simulink model "WholeSystemSimulation"  (R2024b)
settings: Solver=FixedStepAuto  StartTime=0.0  StopTime=3  FixedStep=1/executionRate  MaxStep=0.01  RelTol=1e-3
values from neighbouring files (symbols this model uses):
  executionRate = 5*ADC_SamplingRate    (= 25000)    [parameters.m]
undefined symbols (not defined in the file or in its folder): Batt, VCCS
libraries: fl_lib x15, spsFourierLib x4, nesl_utility x4, simulink_extras x2, ee_lib x1
settings Model: SnapshotBufferSize=100  SnapshotInterval=100  Creator=JesseJabezArendse  LastModifiedBy=JesseJabezArendse
settings SolverCC: MaxConsecutiveMinStep=1000  ShapePreserveControl=EnableAll  ZeroCrossControl=EnableAll  ZeroCrossAlgorithm=Adaptive
settings DebuggingCC: MaskedZcDiagnostic=none  IgnoredZcDiagnostic=none
settings RTWCC: GPUComputeCapability=3.5
settings SimscapeCC: ExplicitSolverDiagnosticOptions=none  SimscapeCompileComponentReuse=on

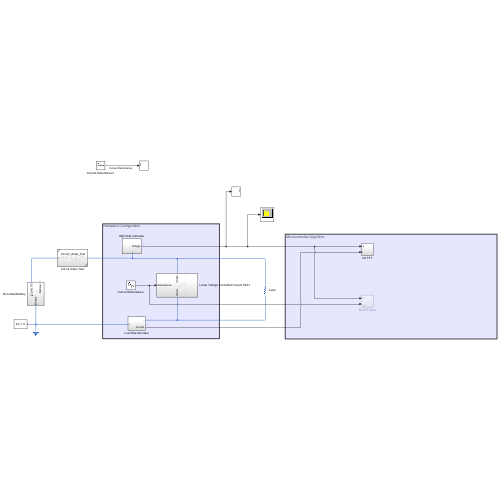
[thumbnail: Simulink's stored preview of the top-level diagram]
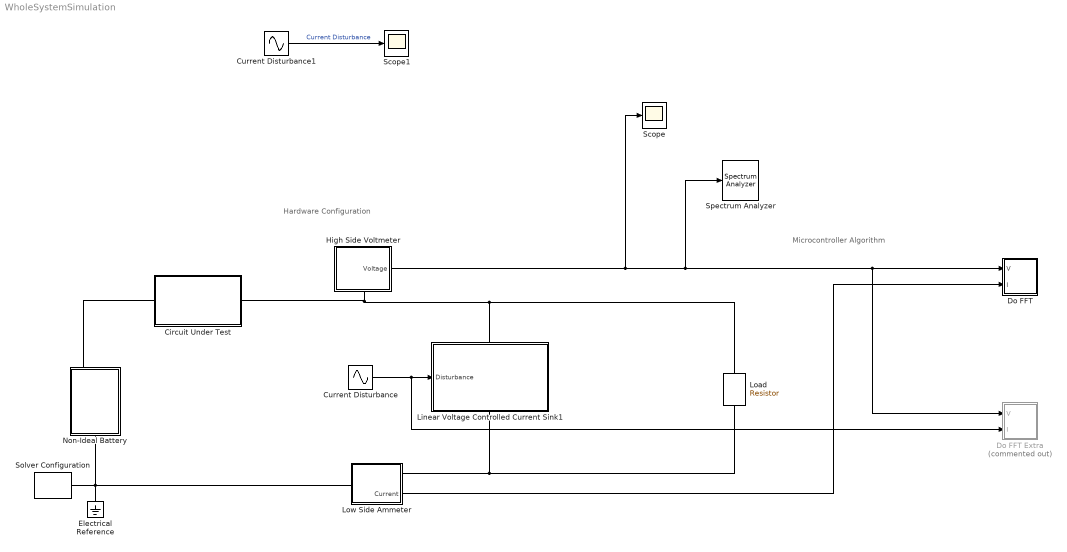
== system WholeSystemSimulation ==
  note: Microcontroller Algorithm
  note: Hardware Configuration
  Circuit Under Test : Subsystem  ReferencedSubsystem=Circuit_Under_Test
  Current Disturbance : Sin  Amplitude=VCCS.Ic/2  Bias=VCCS.Ic/2  Frequency=2*pi*1000  SampleTime=0
  Current Disturbance1 : Sin  Amplitude=VCCS.Ic/2  Bias=VCCS.Ic/2  Frequency=2*pi*1  Phase=-pi/2  SampleTime=0
  Do FFT : Subsystem
  Do FFT Extra : Subsystem  Commented=on
  Electrical Reference : fl_lib/Electrical/Electrical Elements/Electrical Reference
  High Side Voltmeter : Subsystem
      settings: PortSchema="{\"entries\":[{\"content\":{\"sides\":[{\"content\":{\"connectorIds\":[\"LConn1\"]},\"type\":\"ConnectorPlacement.EquallySpacedRectSide\",\"uuid\":\"dc1b0a43-9892-4e76-b578-c6766fff3160\"},{\"content\":{\"side\":\"RIGHT\"},\"type\":\"ConnectorPlacement.EquallySpacedRectSide\",\"uuid\":\"9def735b-7f91-462a-b4cf-02dbc37cb50d\"},{\"content\":{\"connectorIds\":[\"Out1\"],\"side\":\"TOP\"},\"type\":\"ConnectorPlacement.EquallySpacedRectSide\",\"uuid\":\"48b0b69b-e7ce-41ab-9991-9433c11ca6b3\"}]},\"type\":\"ConnectorPlacement.EquallySpacedConnector\",\"uuid\":\"81e0c23a-938e-4893-99ad-7cd29a79d819\"}],\"packageUris\":[\"http://schema.mathworks.com/mf0/Connector/R2020b\"],\"version\":\"1.0\"}"
  Linear Voltage Controlled Current Sink1 : Subsystem
      settings: PortSchema="{\"entries\":[{\"content\":{\"sides\":[{\"content\":{\"connectorIds\":[\"In1\"]},\"type\":\"ConnectorPlacement.EquallySpacedRectSide\",\"uuid\":\"18d529a9-1cf8-4422-88d7-d8552fbc69b1\"},{\"content\":{\"side\":\"RIGHT\"},\"type\":\"ConnectorPlacement.EquallySpacedRectSide\",\"uuid\":\"d099dce7-fb34-4cde-a1aa-9938a0a6f030\"},{\"content\":{\"connectorIds\":[\"LConn1\"],\"side\":\"TOP\"},\"type\":\"ConnectorPlacement.EquallySpacedRectSide\",\"uuid\":\"f8047e6b-d66f-4a7e-8493-e8033d6b44b9\"},{\"content\":{\"connectorIds\":[\"RConn1\"],\"side\":\"BOTTOM\"},\"type\":\"ConnectorPlacement.EquallySpacedRectSide\",\"uuid\":\"82df79ce-b48a-4c65-8b98-c5c94047aaf0\"}]},\"type\":\"ConnectorPlacement.EquallySpacedConnector\",\"uuid\":\"b1df41be-ee9b-457e-b8ab-8cc4e6bfe837\"}],\"packageUris\":[\"http://schema.mathworks.com/mf0/Connector/R2020b\"],\"version\":\"1.0\"}"
  Load : fl_lib/Electrical/Electrical Elements/Resistor  R=15 Ohm  i_specify=off  i_priority=None  i=0 A  i_nominal_specify=off  i_nominal_value=1  i_nominal_unit=A  v_specify=off  v_priority=None  v=0 V  v_nominal_specify=off  v_nominal_value=1  v_nominal_unit=V
  Low Side Ammeter : Subsystem
      settings: PortSchema="{\"entries\":[{\"content\":{\"sides\":[{\"content\":{\"connectorIds\":[\"LConn1\"]},\"type\":\"ConnectorPlacement.EquallySpacedRectSide\",\"uuid\":\"b46022f5-6657-4f49-902e-44a46ebfa2aa\"},{\"content\":{\"connectorIds\":[\"RConn1\",\"Out1\"],\"side\":\"RIGHT\"},\"type\":\"ConnectorPlacement.EquallySpacedRectSide\",\"uuid\":\"78fe3371-6c6c-498b-a57a-7222f53b6f75\"},{\"content\":{\"side\":\"TOP\"},\"type\":\"ConnectorPlacement.EquallySpacedRectSide\",\"uuid\":\"f620f906-e4ba-4bb0-90eb-5c83cecaa9b0\"}]},\"type\":\"ConnectorPlacement.EquallySpacedConnector\",\"uuid\":\"c8c374b0-8252-47d0-a7d3-288c91bf26d8\"}],\"packageUris\":[\"http://schema.mathworks.com/mf0/Connector/R2020b\"],\"version\":\"1.0\"}"
  Non-Ideal Battery : Subsystem
  Scope : Scope
  Scope1 : Scope
  Solver Configuration : nesl_utility/Solver Configuration  PhysicalDomain=network_engine_domain  SubClassName=solver  LeftPortType=input  RightPortType=generic  Tones=[]  Harmonics=[]  SimulateNoise=off  Profile=off  UseLocalSampling=off  EnableSwitchedLinearOptims=on  FrequencyDomain=off  UseCCode=off  RelTol=0.001  AbsTol=0.001  MinStep=1e-09  ToWorkspace=off  RevertToSquareIcSolve=off  NumHomotopyIterations=100  PhasorMode=off  PhasorModeNumHarmonics=1  ConsistencySolver=NEWTON_XTOL_AFTER_FTOL  IndexReductionMethod=None  DoDC=on  ResidualTolerance=1e-09  ConsistencyTolSource=LOCAL  ConsistencyAbsTol=0.001  ConsistencyRelTol=0.001  ConsistencyTolFactor=0.00001  UseLocalSolver=on  LocalSolverChoice=NE_BACKWARD_EULER_ADVANCER  ResolveIndetEquations=on  FunctionEvalNumThread=1  LocalSolverSampleTime=1/executionRate  DoFixedCost=off  MaxNonlinIter=3  MaxModeIter=2  ComputeImpulses=off  ImpulseIterations=2  LinearAlgebra=auto  LinearAlgebraNumThread=0  EquationFormulation=NE_TIME_EF  DelaysMemoryBudget=1024  AutomaticFiltering=off  FilteringTimeConstant=0.001  PartitionStorageMethod=AS_NEEDED  PartitionMemoryBudget=1024  PartitionMethod=ROBUST  MultibodyUseLocalSolver=off  MultibodyLocalSolverChoice=ODE1  MultibodyLocalSolverSampleTime=0.001
  Spectrum Analyzer : SpectrumAnalyzer  WindowPosition=[-276.000000,-288.000000,1536.000000,792.000000,]  ScopeFrameLocation=window  SampleRateSource=Property  SampleRate=50000  WindowInvariantSamplesPerUpdate=on  Span=50000  StartFrequency=-25000  StopFrequency=25000  YLimits=[-122.6326188,59.51523193]  ShowLegend=on
  wires:
  Current Disturbance/1 -> Do FFT Extra/2(I), Linear Voltage Controlled Current Sink1/1(Disturbance)
  High Side Voltmeter/1(Voltage) -> Scope/1, Spectrum Analyzer/1, Do FFT Extra/1(V), Do FFT/1(V)
  Low Side Ammeter/1(Current) -> Do FFT/2(I)
  Current Disturbance1/1 -> Scope1/1  "Current Disturbance"
  connections:
  Solver Configuration/RConn1 -- Low Side Ammeter/LConn1 -- Non-Ideal Battery/RConn1 -- Electrical Reference/LConn1
  High Side Voltmeter/LConn1 -- Linear Voltage Controlled Current Sink1/LConn1 -- Load/LConn1 -- Circuit Under Test/RConn1
  Low Side Ammeter/RConn1 -- Linear Voltage Controlled Current Sink1/RConn1 -- Load/RConn1
  Non-Ideal Battery/LConn1 -- Circuit Under Test/LConn1

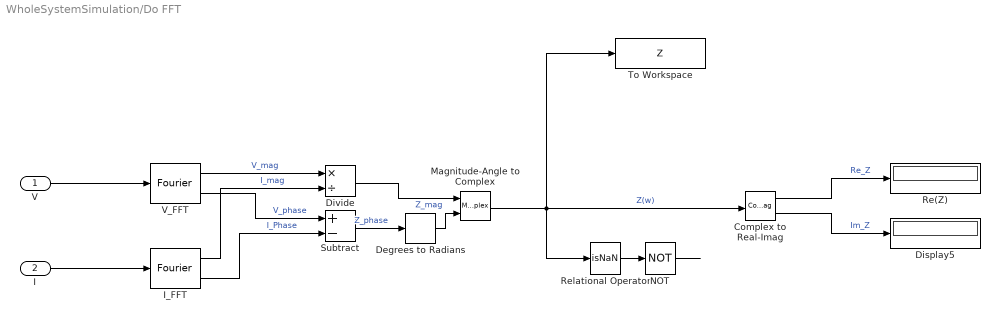
== system WholeSystemSimulation/Do FFT ==
  V : Inport
  I : Inport  Port=2
  Complex to Real-Imag : ComplexToRealImag
  Degrees to Radians : simulink_extras/Transformations/Degrees to Radians
  Display5 : Display
  Divide : Product  Inputs=*/
  I_FFT : spsFourierLib/Fourier  Freq=selectedFreq  n=1  InInit=[0, 0]  Ts=0
  Magnitude-Angle to Complex : MagnitudeAngleToComplex
  NOT : Logic  Operator=NOT  IconShape=distinctive  AllPortsSameDT=off  OutDataTypeStr=boolean
  Re(Z) : Display
  Relational Operator : RelationalOperator  Operator=isNaN  OutDataTypeStr=boolean  RndMeth=Simplest  InputSameDT=off
  Subtract : Sum  Inputs=+-
  To Workspace : ToWorkspace  VariableName=Z  SampleTime=-1
  V_FFT : spsFourierLib/Fourier  Freq=selectedFreq  n=1  InInit=[0, 0]  Ts=0
  wires:
  V_FFT/1 -> Divide/1  "V_mag"
  Degrees to Radians/1 -> Magnitude-Angle to Complex/2
  Magnitude-Angle to Complex/1 -> To Workspace/1, Complex to Real-Imag/1, Relational Operator/1  "Z(w)"
  Complex to Real-Imag/1 -> Re(Z)/1  "Re_Z"
  V_FFT/2 -> Subtract/1  "V_phase"
  I_FFT/2 -> Subtract/2  "I_Phase"
  Complex to Real-Imag/2 -> Display5/1  "Im_Z"
  Subtract/1 -> Degrees to Radians/1  "Z_phase"
  I_FFT/1 -> Divide/2  "I_mag"
  Divide/1 -> Magnitude-Angle to Complex/1  "Z_mag"
  I/1 -> I_FFT/1
  V/1 -> V_FFT/1
  Relational Operator/1 -> NOT/1
  NOT/1 -> ?

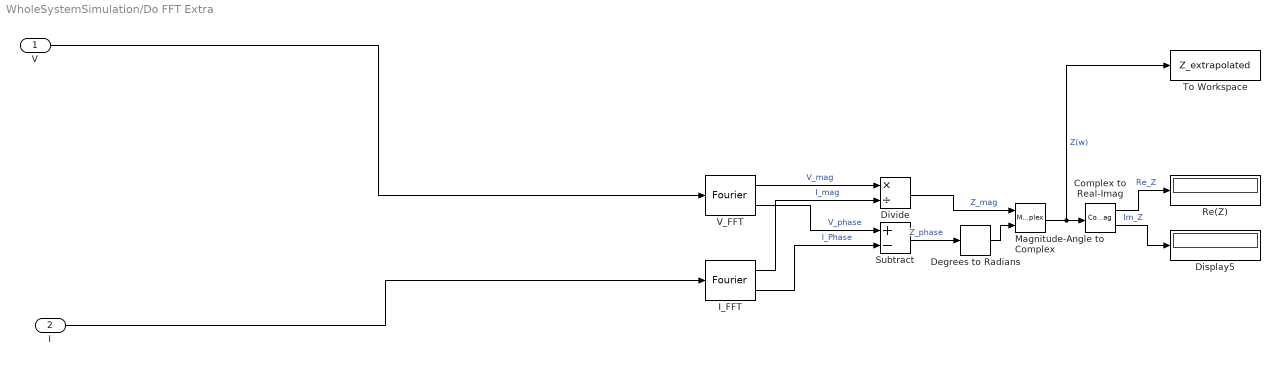
== system WholeSystemSimulation/Do FFT Extra ==
  V : Inport
  I : Inport  Port=2
  Complex to Real-Imag : ComplexToRealImag
  Degrees to Radians : simulink_extras/Transformations/Degrees to Radians
  Display5 : Display
  Divide : Product  Inputs=*/
  I_FFT : spsFourierLib/Fourier  Freq=selectedFreq  n=1  InInit=[0, 0]  Ts=0
  Magnitude-Angle to Complex : MagnitudeAngleToComplex
  Re(Z) : Display
  Subtract : Sum  Inputs=+-
  To Workspace : ToWorkspace  VariableName=Z_extrapolated  SampleTime=-1
  V_FFT : spsFourierLib/Fourier  Freq=selectedFreq  n=1  InInit=[0, 0]  Ts=0
  wires:
  V/1 -> V_FFT/1
  I/1 -> I_FFT/1
  Divide/1 -> Magnitude-Angle to Complex/1  "Z_mag"
  I_FFT/1 -> Divide/2  "I_mag"
  Subtract/1 -> Degrees to Radians/1  "Z_phase"
  Complex to Real-Imag/2 -> Display5/1  "Im_Z"
  I_FFT/2 -> Subtract/2  "I_Phase"
  V_FFT/2 -> Subtract/1  "V_phase"
  Complex to Real-Imag/1 -> Re(Z)/1  "Re_Z"
  Magnitude-Angle to Complex/1 -> Complex to Real-Imag/1, To Workspace/1  "Z(w)"
  Degrees to Radians/1 -> Magnitude-Angle to Complex/2
  V_FFT/1 -> Divide/1  "V_mag"

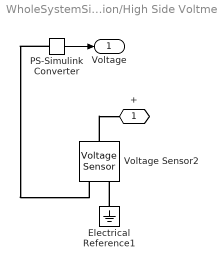
== system WholeSystemSimulation/High Side Voltmeter ==
  Electrical Reference1 : fl_lib/Electrical/Electrical Elements/Electrical Reference
  PS-Simulink Converter : nesl_utility/PS-Simulink Converter  PhysicalDomain=network_engine_domain  SubClassName=ps_output  LeftPortType=input  RightPortType=output  PseudoPeriodic=off  Frequencies=[]  VectorFormat=inherit  Unit=inherit  AffineConversion=off
  Voltage Sensor2 : fl_lib/Electrical/Electrical Sensors/Voltage Sensor
  + : PMIOPort  Side=Left
  Voltage : Outport
  wires:
  PS-Simulink Converter/1 -> Voltage/1
  connections:
  Electrical Reference1/LConn1 -- Voltage Sensor2/RConn2
  PS-Simulink Converter/LConn1 -- Voltage Sensor2/RConn1
  Voltage Sensor2/LConn1 -- +/RConn1

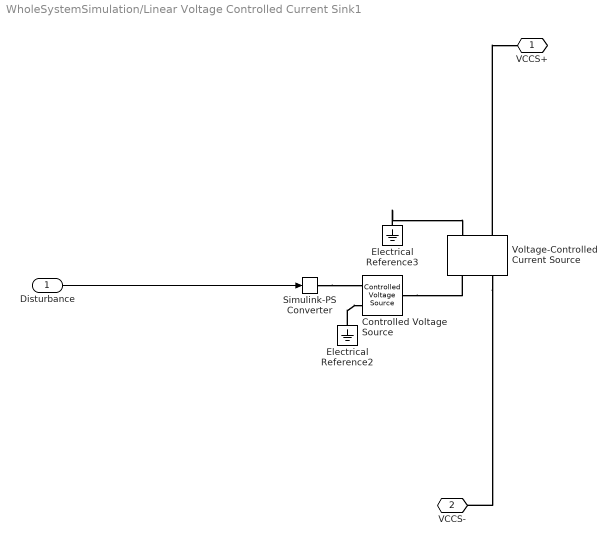
== system WholeSystemSimulation/Linear Voltage Controlled Current Sink1 ==
  Disturbance : Inport
  Controlled Voltage Source : fl_lib/Electrical/Electrical Sources/Controlled Voltage Source
  Electrical Reference2 : fl_lib/Electrical/Electrical Elements/Electrical Reference
  Electrical Reference3 : fl_lib/Electrical/Electrical Elements/Electrical Reference
  Simulink-PS Converter : nesl_utility/Simulink-PS Converter  PhysicalDomain=network_engine_domain  SubClassName=ps_input  LeftPortType=input  RightPortType=output  PseudoPeriodic=off  Frequencies=[]  NoiseDistribution=none  NoiseParameters=[]  Unit=1  AffineConversion=off  FilteringAndDerivatives=provide  SimscapeFilterOrder=1  InputFilterTimeConstant=0.001  UdotUserProvided=0
  Voltage-Controlled Current Source : fl_lib/Electrical/Electrical Sources/Voltage-Controlled Current Source  K=1 1/Ohm  v1_specify=off  v1_priority=None  v1=0 V  v1_nominal_specify=off  v1_nominal_value=1  v1_nominal_unit=V  i2_specify=off  i2_priority=None  i2=0 A  i2_nominal_specify=off  i2_nominal_value=1  i2_nominal_unit=A
      settings: InternalSimscapePortConfiguration="{\"Bottom\":[],\"Left\":[{\"id\":\"p1\",\"label\":\"+\",\"type\":\"foundation.electrical.electrical\"},{\"id\":\"head\",\"label\":\"\",\"type\":\"foundation.electrical.electrical\"}],\"Right\":[{\"id\":\"n1\",\"label\":\"-\",\"type\":\"foundation.electrical.electrical\"},{\"id\":\"tail\",\"label\":\"\",\"type\":\"foundation.electrical.electrical\"}],\"Top\":[]}"
  VCCS+ : PMIOPort  Side=Left
  VCCS- : PMIOPort  Port=2  Side=Right
  wires:
  Disturbance/1 -> Simulink-PS Converter/1
  connections:
  Electrical Reference2/LConn1 -- Controlled Voltage Source/RConn2
  Voltage-Controlled Current Source/RConn2 -- VCCS+/RConn1
  Voltage-Controlled Current Source/LConn2 -- VCCS-/RConn1
  Simulink-PS Converter/RConn1 -- Controlled Voltage Source/RConn1
  Electrical Reference3/LConn1 -- Voltage-Controlled Current Source/RConn1
  Controlled Voltage Source/LConn1 -- Voltage-Controlled Current Source/LConn1

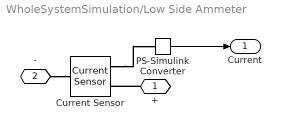
== system WholeSystemSimulation/Low Side Ammeter ==
  Current Sensor : fl_lib/Electrical/Electrical Sensors/Current Sensor
  PS-Simulink Converter : nesl_utility/PS-Simulink Converter  PhysicalDomain=network_engine_domain  SubClassName=ps_output  LeftPortType=input  RightPortType=output  PseudoPeriodic=off  Frequencies=[]  VectorFormat=inherit  Unit=inherit  AffineConversion=off
  + : PMIOPort  Side=Left
  - : PMIOPort  Port=2  Side=Right
  Current : Outport
  wires:
  PS-Simulink Converter/1 -> Current/1
  connections:
  Current Sensor/RConn1 -- PS-Simulink Converter/LConn1
  +/RConn1 -- Current Sensor/RConn2
  -/RConn1 -- Current Sensor/LConn1

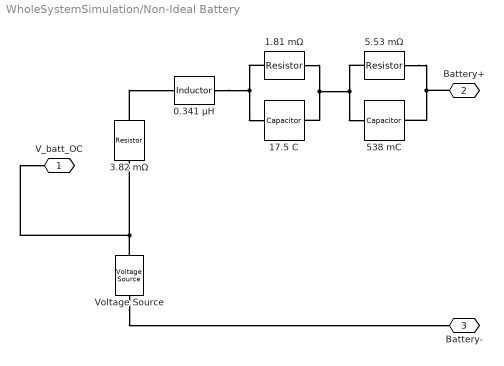
== system WholeSystemSimulation/Non-Ideal Battery ==
  0.341 µH : fl_lib/Electrical/Electrical Elements/Inductor  l=Batt.L_R H  r=0 Ohm  g=0 1/Ohm  i_specify=off  i_priority=None  i=0 A  i_nominal_specify=off  i_nominal_value=1  i_nominal_unit=A  v_specify=off  v_priority=None  v=0 V  v_nominal_specify=off  v_nominal_value=1  v_nominal_unit=V  i_L_specify=off  i_L_priority=High  i_L=0 A  i_L_nominal_specify=off  i_L_nominal_value=1  i_L_nominal_unit=A
  1.81 mΩ : fl_lib/Electrical/Electrical Elements/Resistor  R=Batt.R_1 Ohm  i_specify=off  i_priority=None  i=0 A  i_nominal_specify=off  i_nominal_value=1  i_nominal_unit=A  v_specify=off  v_priority=None  v=0 V  v_nominal_specify=off  v_nominal_value=1  v_nominal_unit=V
  17.5 C : fl_lib/Electrical/Electrical Elements/Capacitor  c=Batt.C_1 F  r=0 Ohm  g=0 1/Ohm  i_specify=off  i_priority=None  i=0 A  i_nominal_specify=off  i_nominal_value=1  i_nominal_unit=A  v_specify=off  v_priority=None  v=0 V  v_nominal_specify=off  v_nominal_value=1  v_nominal_unit=V  vc_specify=off  vc_priority=High  vc=0 V  vc_nominal_specify=off  vc_nominal_value=1  vc_nominal_unit=V
  3.82 mΩ : fl_lib/Electrical/Electrical Elements/Resistor  R=Batt.R_0 Ohm  i_specify=off  i_priority=None  i=0 A  i_nominal_specify=off  i_nominal_value=1  i_nominal_unit=A  v_specify=off  v_priority=None  v=0 V  v_nominal_specify=off  v_nominal_value=1  v_nominal_unit=V
  5.53 mΩ : fl_lib/Electrical/Electrical Elements/Resistor  R=Batt.R_2 Ohm  i_specify=off  i_priority=None  i=0 A  i_nominal_specify=off  i_nominal_value=1  i_nominal_unit=A  v_specify=off  v_priority=None  v=0 V  v_nominal_specify=off  v_nominal_value=1  v_nominal_unit=V
  538 mC : fl_lib/Electrical/Electrical Elements/Capacitor  c=Batt.C_2 F  r=0 Ohm  g=0 1/Ohm  i_specify=off  i_priority=None  i=0 A  i_nominal_specify=off  i_nominal_value=1  i_nominal_unit=A  v_specify=off  v_priority=None  v=0 V  v_nominal_specify=off  v_nominal_value=1  v_nominal_unit=V  vc_specify=off  vc_priority=High  vc=0 V  vc_nominal_specify=off  vc_nominal_value=1  vc_nominal_unit=V
  Voltage Source : ee_lib/Sources/Voltage Source  dc_voltage=Batt.OCV V  ac_voltage=0 V  ac_shift=0 rad  ac_frequency=60 Hz  noise_mode=ee.enum.sources.noise.Disabled  PSD=0 V^2/Hz  sample_time=1e-3 s  repeatability=ee.enum.sources.repeatability.NotRepeatable  user_seed=0  auto_seed=1799798717  i_specify=off  i_priority=None  i=0 A  i_nominal_specify=off  i_nominal_value=1  i_nominal_unit=A  v_specify=off  v_priority=None  v=0 V  v_nominal_specify=off  v_nominal_value=1  v_nominal_unit=V
  V_batt_OC : PMIOPort  Side=Left
  Battery+ : PMIOPort  Port=2  Side=Left
  Battery- : PMIOPort  Port=3  Side=Right
  connections:
  Voltage Source/LConn1 -- V_batt_OC/RConn1 -- 3.82 mΩ/LConn1
  Voltage Source/RConn1 -- Battery-/RConn1
  3.82 mΩ/RConn1 -- 0.341 µH/LConn1
  0.341 µH/RConn1 -- 1.81 mΩ/LConn1 -- 17.5 C/LConn1
  1.81 mΩ/RConn1 -- 538 mC/LConn1 -- 5.53 mΩ/LConn1 -- 17.5 C/RConn1
  5.53 mΩ/RConn1 -- Battery+/RConn1 -- 538 mC/RConn1
